simulink model "int_crit"  (R2025b)
settings: Solver=ode45  StartTime=0.0  StopTime=10.0  RelTol=1e-3  EnableMultiTasking=on
undefined symbols (not defined in the file or in its folder): q_de, q_du, q_u
settings Model: Creator=oravec  LastModifiedBy=juroo
settings SolverCC: AlgebraicLoopSolver=TrustRegion
settings DataIOCC: LimitDataPoints=on  SaveFormat=Array  SignalLoggingSaveFormat=ModelDataLogs  ReturnWorkspaceOutputs=off
settings OptimizationCC: LifeSpan=inf
settings DebuggingCC: SaveWithParameterizedLinksMsg=none  UnderspecifiedInitializationDetection=Classic  MergeDetectMultiDrivingBlocksExec=none  SolverPrmCheckMsg=warning  FcnCallInpInsideContextMsg=warning  UnconnectedInputMsg=warning  UnconnectedOutputMsg=warning  UnconnectedLineMsg=warning  SFUnexpectedBacktrackingDiag=warning  SFNoUnconditionalDefaultTransitionDiag=warning  SFExecutionAtInitializationDiag=none  ArithmeticOperatorsInVariantConditions=warning
settings HardwareCC: ProdBitPerPointer=32.0  ProdBitPerSizeT=32.0  ProdBitPerPtrDiffT=32.0  ProdLargestAtomicFloat=None  ProdIntDivRoundTo=Undefined  ProdEndianess=Unspecified  ProdWordSize=32.0  ProdHWDeviceType=32-bit Generic  TargetHWDeviceType=32-bit Generic
settings ModelReferenceCC: EnableRefExpFcnMdlSchedulingChecks=on  PropagateSignalLabelsOutOfModel=off
settings RTWCC: GPUComputeCapability=3.5  DLArmComputeVersion=19.05
settings CodeAppCC: StateflowObjectComments=on
settings GRTTargetCC: TargetFcnLib=ansi_tfl_tmw.mat  TargetLangStandard=C89/C90 (ANSI)  CombineOutputUpdateFcns=off  GRTInterface=on
settings ConfigComp: CovMetricSettings=dw  CovSaveCumulativeToWorkspaceVar=on  CovSaveSingleToWorkspaceVar=on

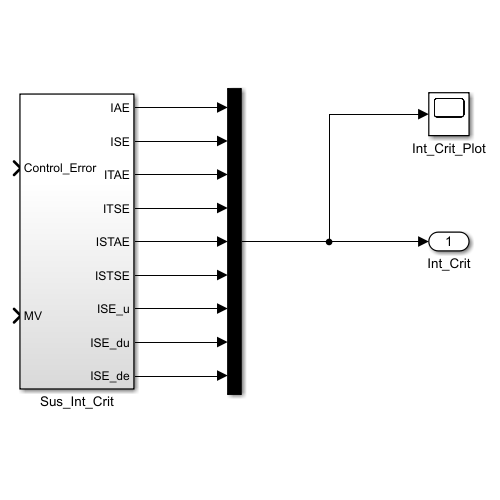
[thumbnail: Simulink's stored preview of the top-level diagram]
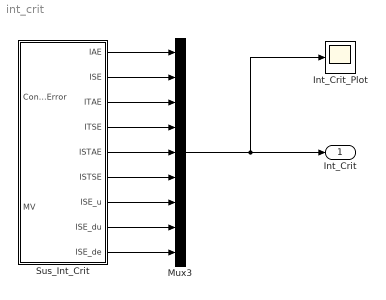
== system int_crit ==
  Int_Crit_Plot : Scope
  Mux3 : Mux  Inputs=9
  Sus_Int_Crit : Subsystem
  Int_Crit : Outport
  wires:
  Sus_Int_Crit/1(IAE) -> Mux3/1
  Sus_Int_Crit/3(ITAE) -> Mux3/3
  Sus_Int_Crit/4(ITSE) -> Mux3/4
  Sus_Int_Crit/5(ISTAE) -> Mux3/5
  Sus_Int_Crit/6(ISTSE) -> Mux3/6
  Sus_Int_Crit/7(ISE_u) -> Mux3/7
  Sus_Int_Crit/8(ISE_du) -> Mux3/8
  Sus_Int_Crit/9(ISE_de) -> Mux3/9
  Mux3/1 -> Int_Crit/1, Int_Crit_Plot/1
  Sus_Int_Crit/2(ISE) -> Mux3/2

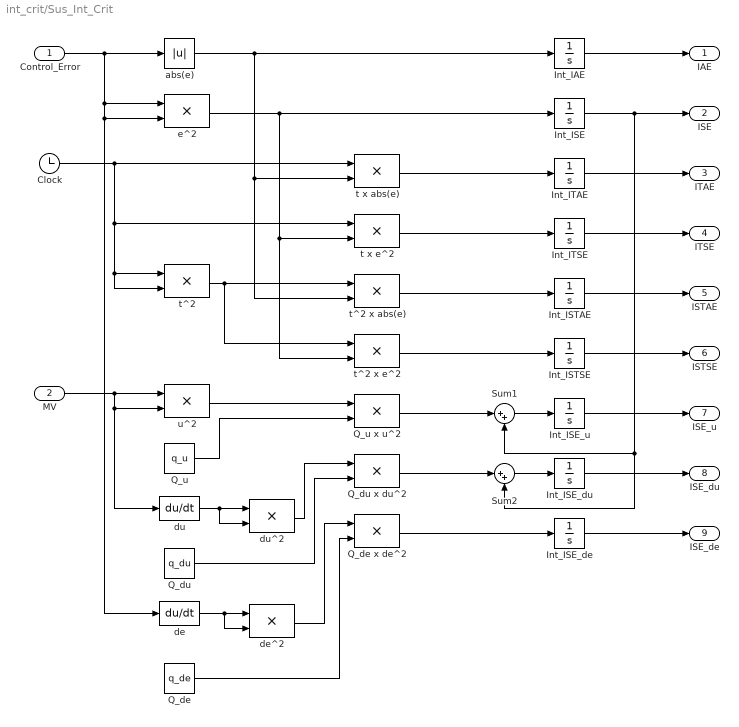
== system int_crit/Sus_Int_Crit ==
  Control_Error : Inport
  MV : Inport  Port=2
  Clock : Clock
  Int_IAE : Integrator
  Int_ISE : Integrator
  Int_ISE_de : Integrator
  Int_ISE_du : Integrator
  Int_ISE_u : Integrator
  Int_ISTAE : Integrator
  Int_ISTSE : Integrator
  Int_ITAE : Integrator
  Int_ITSE : Integrator
  Q_de : Constant  Value=q_de
  Q_de x de^2 : Product  SaturateOnIntegerOverflow=on  OutDataTypeStr=Inherit: Same as first input
  Q_du : Constant  Value=q_du
  Q_du x du^2 : Product  SaturateOnIntegerOverflow=on  OutDataTypeStr=Inherit: Same as first input
  Q_u : Constant  Value=q_u
  Q_u x u^2 : Product  SaturateOnIntegerOverflow=on  OutDataTypeStr=Inherit: Same as first input
  Sum1 : Sum  Inputs=|++  SaturateOnIntegerOverflow=on
  Sum2 : Sum  Inputs=|++  SaturateOnIntegerOverflow=on
  abs(e) : Abs
  de : Derivative
  de^2 : Product  SaturateOnIntegerOverflow=on  OutDataTypeStr=Inherit: Same as first input
  du : Derivative
  du^2 : Product  SaturateOnIntegerOverflow=on  OutDataTypeStr=Inherit: Same as first input
  e^2 : Product  SaturateOnIntegerOverflow=on  OutDataTypeStr=Inherit: Same as first input
  t x abs(e) : Product  SaturateOnIntegerOverflow=on  OutDataTypeStr=Inherit: Same as first input
  t x e^2 : Product  SaturateOnIntegerOverflow=on  OutDataTypeStr=Inherit: Same as first input
  t^2 : Product  SaturateOnIntegerOverflow=on  OutDataTypeStr=Inherit: Same as first input
  t^2 x abs(e) : Product  SaturateOnIntegerOverflow=on  OutDataTypeStr=Inherit: Same as first input
  t^2 x e^2 : Product  SaturateOnIntegerOverflow=on  OutDataTypeStr=Inherit: Same as first input
  u^2 : Product  SaturateOnIntegerOverflow=on  OutDataTypeStr=Inherit: Same as first input
  IAE : Outport
  ISE : Outport  Port=2
  ITAE : Outport  Port=3
  ITSE : Outport  Port=4
  ISTAE : Outport  Port=5
  ISTSE : Outport  Port=6
  ISE_u : Outport  Port=7
  ISE_du : Outport  Port=8
  ISE_de : Outport  Port=9
  wires:
  Control_Error/1 -> abs(e)/1, e^2/1, e^2/2, de/1
  abs(e)/1 -> Int_IAE/1, t x abs(e)/2, t^2 x abs(e)/2
  e^2/1 -> Int_ISE/1, t x e^2/2, t^2 x e^2/2
  Int_ISE/1 -> Sum1/2, Sum2/2, ISE/1
  t x abs(e)/1 -> Int_ITAE/1
  Clock/1 -> t x abs(e)/1, t x e^2/1, t^2/1, t^2/2
  t x e^2/1 -> Int_ITSE/1
  t^2/1 -> t^2 x abs(e)/1, t^2 x e^2/1
  t^2 x abs(e)/1 -> Int_ISTAE/1
  t^2 x e^2/1 -> Int_ISTSE/1
  Sum1/1 -> Int_ISE_u/1
  MV/1 -> u^2/1, u^2/2, du/1
  u^2/1 -> Q_u x u^2/1
  Q_u/1 -> Q_u x u^2/2
  Q_u x u^2/1 -> Sum1/1
  Sum2/1 -> Int_ISE_du/1
  du/1 -> du^2/1, du^2/2
  du^2/1 -> Q_du x du^2/1
  Q_du/1 -> Q_du x du^2/2
  Q_du x du^2/1 -> Sum2/1
  de/1 -> de^2/1, de^2/2
  de^2/1 -> Q_de x de^2/1
  Q_de/1 -> Q_de x de^2/2
  Q_de x de^2/1 -> Int_ISE_de/1
  Int_IAE/1 -> IAE/1
  Int_ITAE/1 -> ITAE/1
  Int_ITSE/1 -> ITSE/1
  Int_ISTAE/1 -> ISTAE/1
  Int_ISTSE/1 -> ISTSE/1
  Int_ISE_u/1 -> ISE_u/1
  Int_ISE_du/1 -> ISE_du/1
  Int_ISE_de/1 -> ISE_de/1
